simulink model "test_Co_Sim"  (R2022b)
settings: Solver=FixedStepDiscrete  StartTime=0.0  StopTime=10.0  FixedStep=1  RelTol=1e-3
InitFcn:
  | eval('test')
settings Model: Creator=anandh  LastModifiedBy=clarkm
settings SolverCC: AlgebraicLoopSolver=TrustRegion
settings DebuggingCC: UnconnectedInputMsg=warning  UnconnectedOutputMsg=warning  UnconnectedLineMsg=warning  SFMachineParentedDataDiag=warning
settings ModelReferenceCC: EnableRefExpFcnMdlSchedulingChecks=on

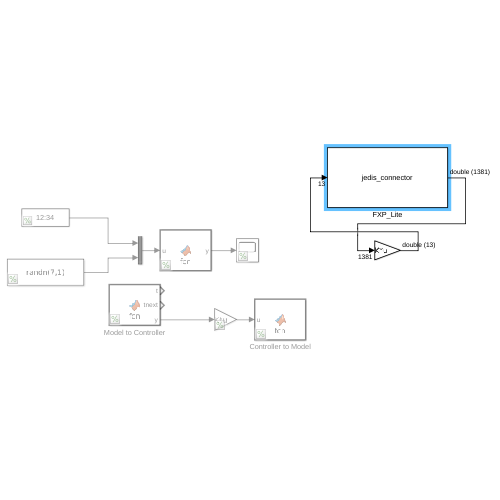
[thumbnail: Simulink's stored preview of the top-level diagram]
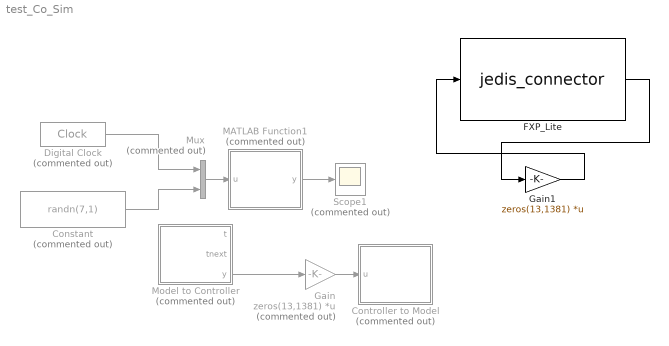
== system test_Co_Sim ==
  Constant : Constant  Commented=on  Value=randn(7,1)
  Controller to Model : MATLAB Function  Commented=on  TreatAsAtomicUnit=on
  Digital Clock : DigitalClock  Commented=on  SampleTime=-1
  FXP_Lite : M-S-Function  FunctionName=jedis_connector
  Gain : Gain  Commented=on  Gain=zeros(13,1381)  Multiplication=Matrix(K*u)
  Gain1 : Gain  Gain=zeros(13,1381)  Multiplication=Matrix(K*u)
  MATLAB Function1 : MATLAB Function  Commented=on  TreatAsAtomicUnit=on
  Model to Controller : MATLAB Function  Commented=on  TreatAsAtomicUnit=on
  Mux : Mux  Commented=on  Inputs=2
  Scope1 : Scope  Commented=on
  wires:
  Model to Controller/3(y) -> Gain/1
  Gain/1 -> Controller to Model/1(u)
  Mux/1 -> MATLAB Function1/1(u)
  Digital Clock/1 -> Mux/1
  Constant/1 -> Mux/2
  MATLAB Function1/1(y) -> Scope1/1
  Gain1/1 -> FXP_Lite/1
  FXP_Lite/1 -> Gain1/1

== matlab function test_Co_Sim/Model to Controller ==
  data: t output; tnext output; y output
function [t,tnext,y] = fcn
% Declare evalin as an extrinsic function
coder.extrinsic('evalin');
coder.extrinsic('jsonencode');
coder.extrinsic('jsondecode');
coder.extrinsic('getfield');

y = zeros(1381,1);
t = 0;
tnext=0;
read_key = 'rdm__state_space_model__pro2req';
timeout = 30;
Out = evalin('base', ['jedis.brpop(' num2str(timeout) ', ''' read_key ''').getValue();']);

Out_json = jsondecode(char(Out));
disp(getfield(Out_json,'y'))
disp("Received y")
y = getfield(Out_json,'y');
t = getfield(Out_json,'t');
tnext = getfield(Out_json,'t_next');

== matlab function test_Co_Sim/Controller to Model ==
  data: u input
function fcn(u)
% Declare evalin as an extrinsic function
coder.extrinsic('evalin');
coder.extrinsic('jsonencode');
coder.extrinsic('jsondecode');
coder.extrinsic('getfield');

write_key = 'rdm__state_space_model__req2pro';
msg_data = jsonencode(struct('u',u));
evalin('base', ['jedis.lpush(''' write_key ''', ''' msg_data ''');']);

== matlab function test_Co_Sim/MATLAB Function1 ==
  data: u input; y output
function y = fcn(u)
% Declare evalin as an extrinsic function
coder.extrinsic('evalin');
coder.extrinsic('jsonencode');
coder.extrinsic('jsondecode');
coder.extrinsic('getfield');

y = zeros(8,1);
key = 'anandh_hello';
msg_data = jsonencode(struct('u',u));
evalin('base', ['jedis.lpush(''' key ''', ''' msg_data ''');']);
timeout = 10;
Out = evalin('base', ['jedis.brpop(' num2str(timeout) ', ''' key ''').getValue();']);
MyArray = getfield(jsondecode(char(Out)),'u');
disp(size(MyArray))
y = MyArray;
